simulink model "opt_model"  (R2021b)
settings: Solver=VariableStepAuto  StartTime=0.0  StopTime=10.0  RelTol=1e-3
InitFcn:
  | load('K.mat')
libraries: cstblocks x1
settings Model: Creator=zafar  LastModifiedBy=zafar

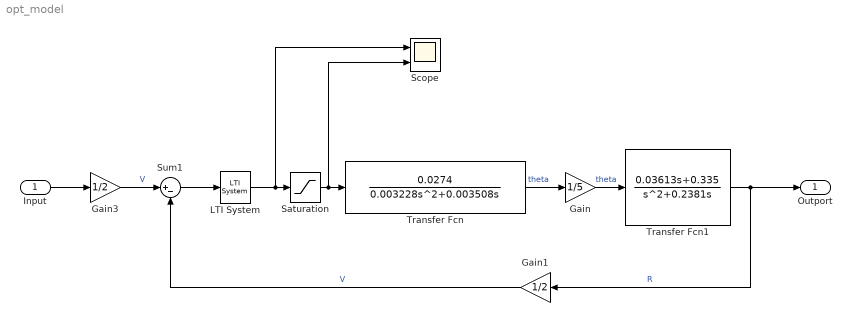
== system opt_model ==
  Input : Inport
  Gain : Gain  Gain=1/5
  Gain1 : Gain  Gain=1/2
  Gain3 : Gain  Gain=1/2
  LTI System : cstblocks/LTI System  sys=K  IC=[]
  Saturation : Saturate  UpperLimit=20  LowerLimit=-20
  Scope : Scope  NumInputPorts=2
  Sum1 : Sum  Inputs=|+-
  Transfer Fcn : TransferFcn  Numerator=[0.0274]  Denominator=[0.003228 0.003508 0]
  Transfer Fcn1 : TransferFcn  Numerator=[0.03613 0.335]  Denominator=[1 0.2381 0]
  Outport : Outport
  wires:
  Gain3/1 -> Sum1/1  "V"
  Gain1/1 -> Sum1/2  "V"
  Transfer Fcn1/1 -> Outport/1, Gain1/1  "R"
  Saturation/1 -> Scope/2, Transfer Fcn/1
  Transfer Fcn/1 -> Gain/1  "theta"
  Gain/1 -> Transfer Fcn1/1  "theta"
  Input/1 -> Gain3/1
  LTI System/1 -> Scope/1, Saturation/1
  Sum1/1 -> LTI System/1
